simulink model "EquivalentCircuit"  (R2022b)
settings: Solver=VariableStepAuto  StartTime=0.0  StopTime=1  RelTol=1e-3
values from neighbouring files (symbols this model uses):
  f = 50    [parameters.m]
  Rc = 1    [parameters.m]
  Rc1 = 1    [parameters.m]
  Rfe = 1    [parameters.m]
  V1 = 200    [parameters.m]
  X1 = 1e-3    (= 0.001)    [parameters.m]
  Xu = 1e-3    (= 0.001)    [parameters.m]
libraries: spsSeriesRLCBranchLib x5, spsACVoltageSourceLib x1, spsCurrentMeasurementLib x1, eePowerMeasurement x1, spsVoltageMeasurementLib x1, spspowerguiLib x1
settings Model: Creator=ramuj  LastModifiedBy=ramuj

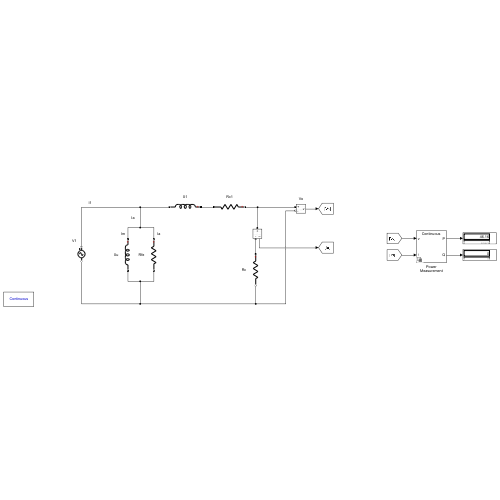
[thumbnail: Simulink's stored preview of the top-level diagram]
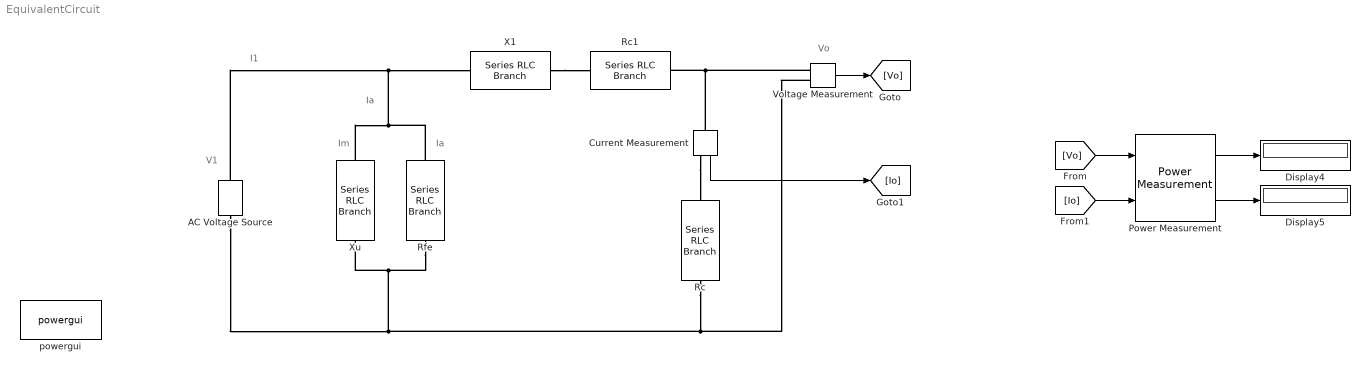
== system EquivalentCircuit ==
  note: Vo
  note: V1
  note: Ia
  note: Im
  note: Ia
  note: I1
  AC Voltage Source : spsACVoltageSourceLib/AC Voltage Source  Amplitude=V1  Phase=0  Frequency=f  SampleTime=0  Measurements=None  BusType=swing  Pref=10e3  Qref=0  Qmin=-inf  Qmax=+inf
  Current Measurement : spsCurrentMeasurementLib/Current Measurement  PhasorSimulation=off  OutputType=Complex  PSBequivalent=0
  Display4 : Display
  Display5 : Display
  Power Measurement : eePowerMeasurement/Power Measurement  LabelModeActiveChoice=Continuous  F=60  K=[0 1 2 3]  Ts=0
  Rc : spsSeriesRLCBranchLib/Series RLC Branch  LConnTagsString=__new0  RConnTagsString=__new0  BranchType=R  Resistance=Rc  Inductance=1e-3  SetiL0=off  InitialCurrent=0  Capacitance=1e-6  Setx0=off  InitialVoltage=0  Measurements=None
  Rc1 : spsSeriesRLCBranchLib/Series RLC Branch  LConnTagsString=__new0  RConnTagsString=__new0  BranchType=R  Resistance=Rc1  Inductance=1e-3  SetiL0=off  InitialCurrent=0  Capacitance=1e-6  Setx0=off  InitialVoltage=0  Measurements=None
  Rfe : spsSeriesRLCBranchLib/Series RLC Branch  LConnTagsString=__new0  RConnTagsString=__new0  BranchType=R  Resistance=Rfe  Inductance=1e-3  SetiL0=off  InitialCurrent=0  Capacitance=1e-6  Setx0=off  InitialVoltage=0  Measurements=None
  Voltage Measurement : spsVoltageMeasurementLib/Voltage Measurement  PhasorSimulation=off  OutputType=Complex  PSBequivalent=0
  X1 : spsSeriesRLCBranchLib/Series RLC Branch  LConnTagsString=__new0  RConnTagsString=__new0  BranchType=L  Resistance=1  Inductance=X1  SetiL0=off  InitialCurrent=0  Capacitance=1e-6  Setx0=off  InitialVoltage=0  Measurements=None
  Xu : spsSeriesRLCBranchLib/Series RLC Branch  LConnTagsString=__new0  RConnTagsString=__new0  BranchType=L  Resistance=1  Inductance=Xu  SetiL0=off  InitialCurrent=0  Capacitance=1e-6  Setx0=off  InitialVoltage=0  Measurements=None
  powergui : spspowerguiLib/powergui  Priority=1  SimulationMode=Continuous  SampleTime=50e-6  frequency=60  Iterations=50  frequencyindice=50  Pbase=100e6  ErrMax=1e-4  UnitsV=kV  UnitsW=MW  buscounter=0  FunctionMessages=off  echomessages=off  EnableUseOfTLC=off  CurrentSourceSwitches=off  DisableSnubberDevices=off  DisableRonSwitches=off  DisableVfSwitches=off  DisplayEquations=off  AutomaticDiscreteSolvers=off  SolverType=Tustin/Backward Euler (TBE)  Interpol=off  ExternalGateDelay=off  methode=off  Ts=100  x0status=blocks  SPID=on  SwTol=0  HookPort=off  NonlinearTolerance=1e-4  nMaxIteration=100  ContinueOnMaxIteration=off  RestoreLinks=warning  ResistiveCurrentMeasurement=off  Frange=[0:2:500]  Ylog=off  Xlog=on  ShowGrid=off  save=off  variable=ZData  structure=0  ZoomFFT=off  StartTime=0.0  cycles=1  DisplayStyle=1  fundamental=60  FreqAxis=off  MaxFrequency=1000  frequencyindicesteady=1  RmsSteady=1  display=off
  wires:
  Voltage Measurement/1 -> [Vo]
  Power Measurement/1 -> Display4/1
  Power Measurement/2 -> Display5/1
  Current Measurement/1 -> [Io]
  [Vo] -> Power Measurement/1
  [Io] -> Power Measurement/2
  connections:
  Rfe/LConn1 -- Xu/LConn1 -- AC Voltage Source/RConn1 -- X1/RConn1
  X1/LConn1 -- Rc1/RConn1
  Voltage Measurement/LConn1 -- Current Measurement/LConn1 -- Rc1/LConn1
  Rc/RConn1 -- Voltage Measurement/LConn2 -- AC Voltage Source/LConn1 -- Xu/RConn1 -- Rfe/RConn1
  Current Measurement/RConn1 -- Rc/LConn1
